simulink model "WindPrototipeN"  (R2019b)
settings: Solver=ode23s  StartTime=0.0  StopTime=Ts  FixedStep=2  RelTol=5
values from neighbouring files (symbols this model uses):
  c1 = 0.51763    [matlab.mat]
  c2 = 116    [matlab.mat]
  c3 = 0.4    [matlab.mat]
  c4 = 5    [matlab.mat]
  c5 = 21    [matlab.mat]
  c6 = 0.006795    [matlab.mat]
  Tp = 2e-05    [matlab.mat]
undefined symbols (not defined in the file or in its folder): Cogent, DiscIntNeverNeededParam, Ion, Kepware, Lithium, localhost, sigbuilder_block
libraries: powerlib x266, powerlib_extras x83, simulink x30, powerlib_meascontrol x13, opclib x11, sldrtlib x8, electricdrivelib x3
(part 1 of 9)
settings Model: SimulationMode=accelerator  NumberOfSteps=100  Creator=cbhende  LastModifiedBy=EK
settings SolverCC: ZeroCrossControl=DisableAll  AutoInsertRateTranBlk=on
settings DataIOCC: LimitDataPoints=on  LoadInitialState=on  SaveFormat=StructureWithTime  SignalLoggingSaveFormat=ModelDataLogs  SaveOutput=off  SignalLogging=off  SaveTime=off  ReturnWorkspaceOutputs=off
settings OptimizationCC: DefaultParameterBehavior=Inlined  ExpressionDepthLimit=2147483647  InitFltsAndDblsToZero=on  EfficientFloat2IntCast=on  LifeSpan=inf
settings DebuggingCC: UnderspecifiedInitializationDetection=Classic  MergeDetectMultiDrivingBlocksExec=none  SolverPrmCheckMsg=warning  MultiTaskRateTransMsg=warning  FcnCallInpInsideContextMsg=warning  StateNameClashWarn=warning  SFUnexpectedBacktrackingDiag=warning  SFNoUnconditionalDefaultTransitionDiag=warning  SFExecutionAtInitializationDiag=none  ArithmeticOperatorsInVariantConditions=warning
settings HardwareCC: ProdBitPerPointer=32  ProdBitPerSizeT=32  ProdBitPerPtrDiffT=32  ProdLargestAtomicFloat=None  ProdIntDivRoundTo=Undefined  ProdEndianess=Unspecified  ProdWordSize=32  ProdHWDeviceType=32-bit Generic
settings ModelReferenceCC: PropagateSignalLabelsOutOfModel=off
settings SFSimCC: SimUseLocalCustomCode=off  CustomCodeUndefinedFunction=UseInterfaceOnly
settings RTWCC: RTWUseLocalCustomCode=off
settings CodeAppCC: StateflowObjectComments=on
settings GRTTargetCC: TargetLangStandard=C89/C90 (ANSI)  GeneratePreprocessorConditionals=Disable all  CombineOutputUpdateFcns=off  GRTInterface=on
settings ConfigComp: CovMetricSettings=dw  CovHtmlReporting=on  CovSaveCumulativeToWorkspaceVar=on  CovSaveSingleToWorkspaceVar=on  CovExternalEMLEnable=off

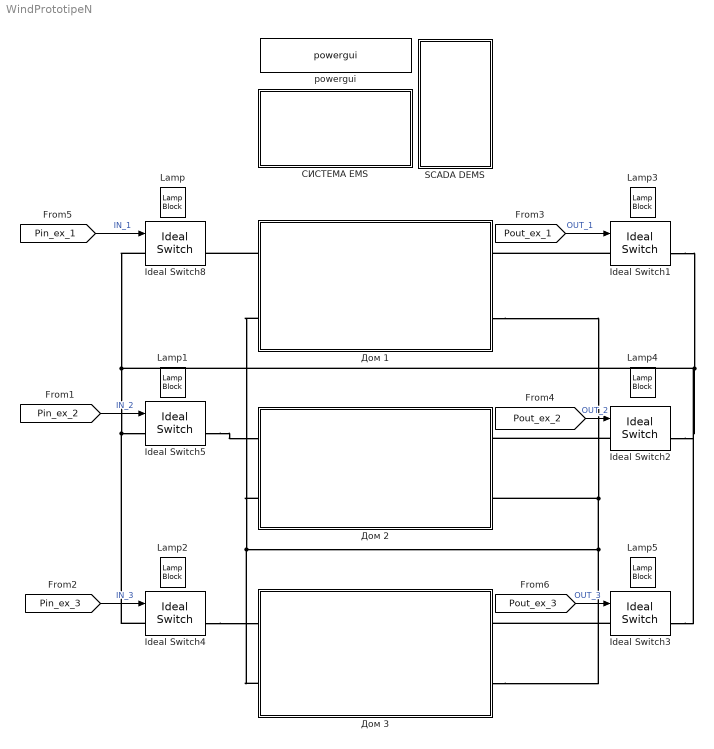
== system WindPrototipeN ==
  Ideal Switch{1..5,8} (6 alike) : powerlib/Power Electronics/Ideal Switch  Ron=0.001  Lon=0  IC=0  Rs=1e5  Cs=inf  Measurements=on
      settings: SourceProductName=Simscape Electrical
  Lamp{,1..5} (6 alike) : LampBlock
  SCADA DEMS : Subsystem
  powergui : powerlib/powergui  Priority=1  SimulationMode=Discrete  SampleTime=Tp  frequency=60  Iterations=50  frequencyindice=0  Pbase=100e6  ErrMax=1e-4  UnitsV=kV  UnitsW=MW  buscounter=0  FunctionMessages=off  echomessages=off  EnableUseOfTLC=off  CurrentSourceSwitches=off  DisableSnubberDevices=off  DisableRonSwitches=off  DisableVfSwitches=off  DisplayEquations=off  AutomaticDiscreteSolvers=off  SolverType=Tustin/Backward Euler (TBE)  Interpol=off  ExternalGateDelay=off  methode=off  Ts=100  x0status=blocks  SPID=off  SwTol=0  HookPort=off  NonlinearTolerance=1e-4  nMaxIteration=100  ContinueOnMaxIteration=off  RestoreLinks=warning  ResistiveCurrentMeasurement=off  Frange=[0:2:500]  Ylog=off  Xlog=on  ShowGrid=off  save=off  variable=ZData  structure=Generator_Terminal  ZoomFFT=off  StartTime=0.0  cycles=1  DisplayStyle=1  fundamental=50  FreqAxis=off  MaxFrequency=4000  frequencyindicesteady=1  RmsSteady=1  display=off
      settings: SourceProductName=Simscape Electrical
  Дом 1 : Subsystem
  Дом 2 : Subsystem
  Дом 3 : Subsystem
  СИСТЕМА EMS : Subsystem
  wires:
  [Pin_ex_1] -> Ideal Switch8/1  "IN_1"
  [Pin_ex_2] -> Ideal Switch5/1  "IN_2"
  [Pin_ex_3] -> Ideal Switch4/1  "IN_3"
  [Pout_ex_1] -> Ideal Switch1/1  "OUT_1"
  [Pout_ex_2] -> Ideal Switch2/1  "OUT_2"
  [Pout_ex_3] -> Ideal Switch3/1  "OUT_3"
  connections:
  Ideal Switch1/LConn1 -- Дом 1/RConn1
  Ideal Switch2/LConn1 -- Дом 2/RConn1
  Ideal Switch5/RConn1 -- Дом 2/LConn1
  Дом 1/LConn1 -- Ideal Switch8/RConn1
  Ideal Switch4/RConn1 -- Дом 3/LConn1
  Ideal Switch1/RConn1 -- Ideal Switch3/RConn1 -- Ideal Switch2/RConn1 -- Ideal Switch4/LConn1 -- Ideal Switch5/LConn1 -- Ideal Switch8/LConn1
  Дом 3/LConn2 -- Дом 3/RConn2 -- Дом 1/RConn2 -- Дом 2/RConn2 -- Дом 1/LConn2 -- Дом 2/LConn2
  Ideal Switch3/LConn1 -- Дом 3/RConn1

== system WindPrototipeN/SCADA DEMS ==
  note: Доступная мощность ВИЭ
      | всех домов (кВт)
  note: Нагрузка
      | PV WP
      | Мощность общая
      | в сети
  note: Потребление всех домов
  note: Нагрузка
      | PV WP
      | Мощность общая
      | в сети
  note: Нагрузка
      | PV WP
      | Мощность общая
      | в сети
  Display{1..14} (14 alike) : DisplayBlock  LabelPosition=Hide  Format=short  Transparency=1
  OPC : Subsystem
  THINGSPEAK : Subsystem
  Мониторинг матлаб : Subsystem

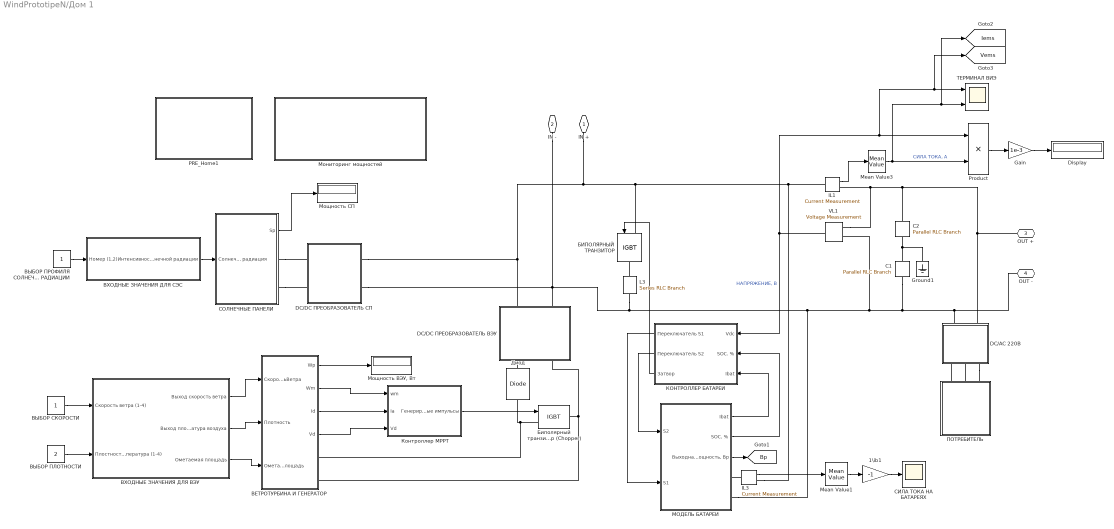
== system WindPrototipeN/Дом 1 ==
  1\ib1 : Gain  Gain=-1  SaturateOnIntegerOverflow=on  OutDataTypeStr=Inherit: Same as input  ParamDataTypeStr=Inherit: Same as input
  C1 : powerlib/Elements/Parallel RLC Branch  LConnTagsString=a  RConnTagsString=__new0  BranchType=C  Resistance=1.0  Inductance=1.0  SetiL0=off  InitialCurrent=0  Capacitance=2200e-06*2  Setx0=off  InitialVoltage=0  Measurements=None
      settings: SourceProductName=Simscape Electrical
  C2 : powerlib/Elements/Parallel RLC Branch  LConnTagsString=a  RConnTagsString=__new0  BranchType=C  Resistance=1.0  Inductance=1.0  SetiL0=off  InitialCurrent=0  Capacitance=2200e-06*2  Setx0=off  InitialVoltage=0  Measurements=None
      settings: SourceProductName=Simscape Electrical
  DC/AC 220В : Subsystem
  DC/DC ПРЕОБРАЗОВАТЕЛЬ ВЭУ : Subsystem
  DC/DC ПРЕОБРАЗОВАТЕЛЬ СП : Subsystem
  Display : Display
  Gain : Gain  Gain=1e-3
  Ground1 : powerlib/Elements/Ground  LConnTagsString=a
      settings: SourceProductName=Simscape Electrical
  IL1 : powerlib/Measurements/Current Measurement  PhasorSimulation=off  OutputType=Complex  PSBequivalent=0
      settings: SourceProductName=Simscape Electrical
  IL3 : powerlib/Measurements/Current Measurement  PhasorSimulation=off  OutputType=Complex  PSBequivalent=0
      settings: SourceProductName=Simscape Electrical
  L3 : powerlib/Elements/Series RLC Branch  LConnTagsString=__new0  RConnTagsString=__new0  BranchType=R  Resistance=19  Inductance=2e-3  SetiL0=off  InitialCurrent=0  Capacitance=1.0  Setx0=off  InitialVoltage=0  Measurements=None
      settings: SourceProductName=Simscape Electrical
  Mean Value1 : powerlib_extras/Measurements/Mean Value  Period=1/110
      settings: SourceProductName=Simscape Electrical  SourceProductBaseCode=PS
  Mean Value3 : powerlib_extras/Measurements/Mean Value  Period=1/110
      settings: SourceProductName=Simscape Electrical  SourceProductBaseCode=PS
  PRE_Home1 : Subsystem
  Product : Product
  VL1 : powerlib/Measurements/Voltage Measurement  Tag=PoWeRsYsTeMmEaSuReMeNt  PhasorSimulation=off  OutputType=Magnitude  PSBequivalent=0
      settings: SourceProductName=Simscape Electrical
  БИПОЛЯРНЫЙ ТРАНЗИТОР : powerlib/Power Electronics/IGBT  Ron=0.001  Lon=0  Vf=1  Tf=1e-6  Tt=2e-6  IC=0  Rs=1e5  Cs=inf  Measurements=off
      settings: SourceProductName=Simscape Electrical
  Биполярный транзистор (Chopper) : powerlib/Power Electronics/IGBT  Ron=0.001  Lon=0  Vf=1  Tf=1e-6  Tt=2e-6  IC=0  Rs=1e5  Cs=inf  Measurements=off
      settings: SourceProductName=Simscape Electrical
  ВЕТРОТУРБИНА И ГЕНЕРАТОР : Subsystem
  ВХОДНЫЕ ЗНАЧЕНИЯ ДЛЯ ВЭУ : Subsystem
  ВХОДНЫЕ ЗНАЧЕНИЯ ДЛЯ СЭС : Subsystem
  ВЫБОР ПЛОТНОСТИ : Constant  Value=2
  ВЫБОР ПРОФИЛЯ СОЛНЕЧНОЙ РАДИАЦИИ : Constant
  ВЫБОР СКОРОСТИ : Constant
  Диод : powerlib/Power Electronics/Diode  Ron=0.01  Lon=0  Vf=0.8  IC=0  UseSnubber=off  Rs=100  Cs=0.1e-6  Measurements=off
      settings: SourceProductName=Simscape Electrical
  КОНТРОЛЛЕР БАТАРЕИ : Subsystem
  Контроллер MPPT : Subsystem
  МОДЕЛЬ БАТАРЕИ : Subsystem
  Мониторинг мощностей : Subsystem
  "Мощность ВЭУ, Вт" : Display
      settings: SampleTime=1e-3
  Мощность СП : Display
      settings: SampleTime=1e-3
  ПОТРЕБИТЕЛЬ : Subsystem
  СИЛА ТОКА НА БАТАРЕЯХ : Scope
  СОЛНЕЧНЫЕ ПАНЕЛИ : Subsystem
  ТЕРМИНАЛ ВИЭ : Scope  NumInputPorts=2
  IN + : PMIOPort  Side=Left
  IN - : PMIOPort  Port=2  Side=Left
  OUT + : PMIOPort  Port=3  Side=Right
  OUT - : PMIOPort  Port=4  Side=Right
  tag scope: Bp=global, Iems=global, Vems=global
  wires:
  1\ib1/1 -> СИЛА ТОКА НА БАТАРЕЯХ/1
  VL1/1 -> КОНТРОЛЛЕР БАТАРЕИ/1(Vdc), [Vems], ТЕРМИНАЛ ВИЭ/1, Product/1  "НАПРЯЖЕНИЕ, В"
  ВЫБОР СКОРОСТИ/1 -> ВХОДНЫЕ ЗНАЧЕНИЯ ДЛЯ ВЭУ/1(Скорость ветра (1-4))
  Mean Value3/1 -> [Iems], ТЕРМИНАЛ ВИЭ/2, Product/2  "СИЛА ТОКА, А"
  МОДЕЛЬ БАТАРЕИ/1(Ibat) -> КОНТРОЛЛЕР БАТАРЕИ/3(Ibat)
  ВХОДНЫЕ ЗНАЧЕНИЯ ДЛЯ ВЭУ/2(Выход плотность и температура воздуха) -> ВЕТРОТУРБИНА И ГЕНЕРАТОР/2(Плотность)
  ВХОДНЫЕ ЗНАЧЕНИЯ ДЛЯ ВЭУ/3(Ометаемая площадь) -> ВЕТРОТУРБИНА И ГЕНЕРАТОР/3(Ометаемая площадь)
  IL1/1 -> Mean Value3/1
  ВЫБОР ПЛОТНОСТИ/1 -> ВХОДНЫЕ ЗНАЧЕНИЯ ДЛЯ ВЭУ/2(Плостность воздуха и температура (1-4))
  IL3/1 -> Mean Value1/1
  Mean Value1/1 -> 1\ib1/1
  ВХОДНЫЕ ЗНАЧЕНИЯ ДЛЯ СЭС/1(Интенсивность солнечной радиации) -> СОЛНЕЧНЫЕ ПАНЕЛИ/1(Солнечная радиация)
  ВХОДНЫЕ ЗНАЧЕНИЯ ДЛЯ ВЭУ/1(Выход скорость ветра) -> ВЕТРОТУРБИНА И ГЕНЕРАТОР/1(СкоростьВетра)
  МОДЕЛЬ БАТАРЕИ/2("SOC, %") -> КОНТРОЛЛЕР БАТАРЕИ/2(SOC. %)
  ВЫБОР ПРОФИЛЯ СОЛНЕЧНОЙ РАДИАЦИИ/1 -> ВХОДНЫЕ ЗНАЧЕНИЯ ДЛЯ СЭС/1(Номер (1,2))
  СОЛНЕЧНЫЕ ПАНЕЛИ/1(Sp) -> Мощность СП/1
  ВЕТРОТУРБИНА И ГЕНЕРАТОР/1(Wp) -> "Мощность ВЭУ, Вт"/1
  Product/1 -> Gain/1
  Gain/1 -> Display/1
  КОНТРОЛЛЕР БАТАРЕИ/2(Переключатель S2) -> МОДЕЛЬ БАТАРЕИ/1(S2)
  КОНТРОЛЛЕР БАТАРЕИ/1(Переключатель S1) -> МОДЕЛЬ БАТАРЕИ/2(S1)
  КОНТРОЛЛЕР БАТАРЕИ/3(Затвор) -> БИПОЛЯРНЫЙ ТРАНЗИТОР/1
  МОДЕЛЬ БАТАРЕИ/3("Выходная мощность, Bp") -> [Bp]
  Контроллер MPPT/1(Генерируемые импульсы) -> Биполярный транзистор (Chopper)/1
  ВЕТРОТУРБИНА И ГЕНЕРАТОР/2(Wm) -> Контроллер MPPT/1(wm)
  ВЕТРОТУРБИНА И ГЕНЕРАТОР/3(Id) -> Контроллер MPPT/2(Ia)
  ВЕТРОТУРБИНА И ГЕНЕРАТОР/4(Vd) -> Контроллер MPPT/3(Vd)
  connections:
  СОЛНЕЧНЫЕ ПАНЕЛИ/RConn2 -- DC/DC ПРЕОБРАЗОВАТЕЛЬ СП/LConn2
  ПОТРЕБИТЕЛЬ/LConn1 -- DC/AC 220В/RConn1
  DC/AC 220В/RConn3 -- ПОТРЕБИТЕЛЬ/LConn3
  Диод/LConn1 -- ВЕТРОТУРБИНА И ГЕНЕРАТОР/RConn1 -- Биполярный транзистор (Chopper)/LConn1
  OUT +/RConn1 -- DC/AC 220В/LConn2 -- C2/LConn1 -- IL1/RConn1 -- VL1/LConn1
  L3/RConn1 -- IN -/RConn1 -- DC/DC ПРЕОБРАЗОВАТЕЛЬ СП/RConn2 -- DC/DC ПРЕОБРАЗОВАТЕЛЬ ВЭУ/RConn2 -- C1/RConn1 -- OUT -/RConn1 -- DC/AC 220В/LConn1 -- VL1/LConn2 -- МОДЕЛЬ БАТАРЕИ/RConn2
  C2/RConn1 -- C1/LConn1 -- Ground1/LConn1
  L3/LConn1 -- БИПОЛЯРНЫЙ ТРАНЗИТОР/RConn1
  ПОТРЕБИТЕЛЬ/LConn2 -- DC/AC 220В/RConn2
  IL3/LConn1 -- МОДЕЛЬ БАТАРЕИ/RConn1
  СОЛНЕЧНЫЕ ПАНЕЛИ/RConn1 -- DC/DC ПРЕОБРАЗОВАТЕЛЬ СП/LConn1
  IL1/LConn1 -- IL3/RConn1 -- DC/DC ПРЕОБРАЗОВАТЕЛЬ ВЭУ/RConn1 -- DC/DC ПРЕОБРАЗОВАТЕЛЬ СП/RConn1 -- IN +/RConn1 -- БИПОЛЯРНЫЙ ТРАНЗИТОР/LConn1
  Биполярный транзистор (Chopper)/RConn1 -- ВЕТРОТУРБИНА И ГЕНЕРАТОР/RConn2 -- DC/DC ПРЕОБРАЗОВАТЕЛЬ ВЭУ/LConn2
  DC/DC ПРЕОБРАЗОВАТЕЛЬ ВЭУ/LConn1 -- Диод/RConn1

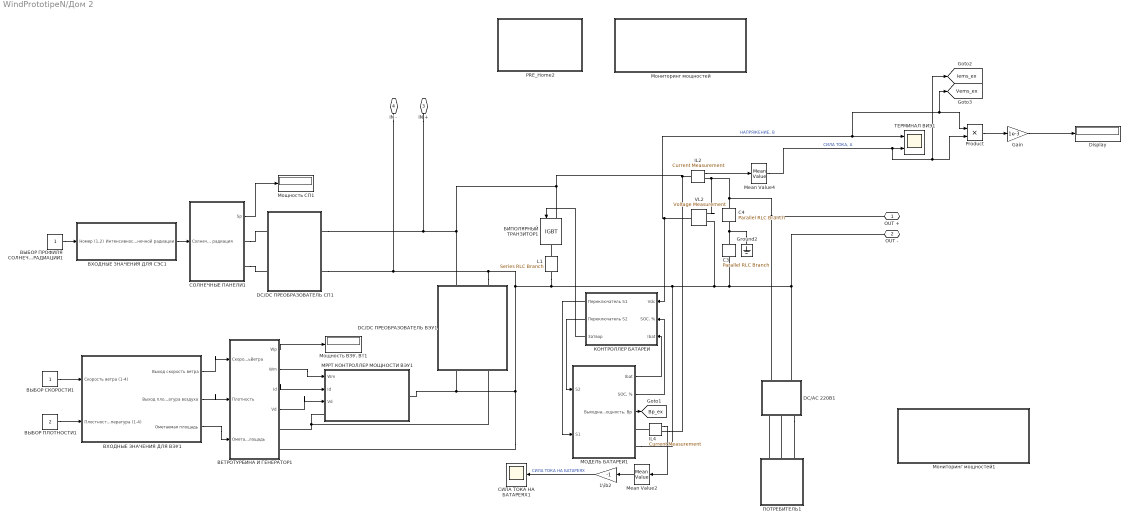
== system WindPrototipeN/Дом 2 ==
  1\ib2 : Gain  Gain=-1  SaturateOnIntegerOverflow=on  OutDataTypeStr=Inherit: Same as input  ParamDataTypeStr=Inherit: Same as input
  C3 : powerlib/Elements/Parallel RLC Branch  LConnTagsString=a  RConnTagsString=__new0  BranchType=C  Resistance=1.0  Inductance=1.0  SetiL0=off  InitialCurrent=0  Capacitance=2200e-06*2  Setx0=off  InitialVoltage=0  Measurements=None
      settings: SourceProductName=Simscape Electrical
  C4 : powerlib/Elements/Parallel RLC Branch  LConnTagsString=a  RConnTagsString=__new0  BranchType=C  Resistance=1.0  Inductance=1.0  SetiL0=off  InitialCurrent=0  Capacitance=2200e-06*2  Setx0=off  InitialVoltage=0  Measurements=None
      settings: SourceProductName=Simscape Electrical
  DC/AC 220В1 : Subsystem
  DC/DC ПРЕОБРАЗОВАТЕЛЬ ВЭУ1 : Subsystem
  DC/DC ПРЕОБРАЗОВАТЕЛЬ СП1 : Subsystem
  Display : Display
  Gain : Gain  Gain=1e-3
  Ground2 : powerlib/Elements/Ground  LConnTagsString=a
      settings: SourceProductName=Simscape Electrical
  IL2 : powerlib/Measurements/Current Measurement  PhasorSimulation=off  OutputType=Complex  PSBequivalent=0
      settings: SourceProductName=Simscape Electrical
  IL4 : powerlib/Measurements/Current Measurement  PhasorSimulation=off  OutputType=Complex  PSBequivalent=0
      settings: SourceProductName=Simscape Electrical
  L1 : powerlib/Elements/Series RLC Branch  LConnTagsString=__new0  RConnTagsString=__new0  BranchType=R  Resistance=19  Inductance=2e-3  SetiL0=off  InitialCurrent=0  Capacitance=1.0  Setx0=off  InitialVoltage=0  Measurements=None
      settings: SourceProductName=Simscape Electrical
  MPPT КОНТРОЛЛЕР МОЩНОСТИ ВЭУ1 : Subsystem
  Mean Value2 : powerlib_extras/Measurements/Mean Value  Period=1/110
      settings: SourceProductName=Simscape Electrical  SourceProductBaseCode=PS
  Mean Value4 : powerlib_extras/Measurements/Mean Value  Period=1/110
      settings: SourceProductName=Simscape Electrical  SourceProductBaseCode=PS
  PRE_Home2 : Subsystem
  Product : Product
  VL2 : powerlib/Measurements/Voltage Measurement  Tag=PoWeRsYsTeMmEaSuReMeNt  PhasorSimulation=off  OutputType=Magnitude  PSBequivalent=0
      settings: SourceProductName=Simscape Electrical
  БИПОЛЯРНЫЙ ТРАНЗИТОР1 : powerlib/Power Electronics/IGBT  Ron=0.001  Lon=0  Vf=1  Tf=1e-6  Tt=2e-6  IC=0  Rs=1e5  Cs=inf  Measurements=off
      settings: SourceProductName=Simscape Electrical
  ВЕТРОТУРБИНА И ГЕНЕРАТОР1 : Subsystem
  ВХОДНЫЕ ЗНАЧЕНИЯ ДЛЯ ВЭУ1 : Subsystem
  ВХОДНЫЕ ЗНАЧЕНИЯ ДЛЯ СЭС1 : Subsystem
  ВЫБОР ПЛОТНОСТИ1 : Constant  Value=2
  ВЫБОР ПРОФИЛЯ СОЛНЕЧНОЙ РАДИАЦИИ1 : Constant
  ВЫБОР СКОРОСТИ1 : Constant
  КОНТРОЛЛЕР БАТАРЕИ : Subsystem
  МОДЕЛЬ БАТАРЕИ1 : Subsystem
  Мониторинг мощностей : Subsystem
  Мониторинг мощностей1 : Subsystem
  "Мощность ВЭУ, Вт1" : Display
      settings: SampleTime=1e-3
  Мощность СП1 : Display
      settings: SampleTime=1e-3
  ПОТРЕБИТЕЛЬ1 : Subsystem
  СИЛА ТОКА НА БАТАРЕЯХ1 : Scope
  СОЛНЕЧНЫЕ ПАНЕЛИ1 : Subsystem
  ТЕРМИНАЛ ВИЭ1 : Scope  NumInputPorts=2
  OUT + : PMIOPort  Side=Right
  OUT - : PMIOPort  Port=2  Side=Right
  IN + : PMIOPort  Port=3  Side=Left
  IN - : PMIOPort  Port=4  Side=Left
  tag scope: Bp_ex=global, Iems_ex=global, Vems_ex=global
  wires:
  1\ib2/1 -> СИЛА ТОКА НА БАТАРЕЯХ1/1  "СИЛА ТОКА НА БАТАРЕЯХ"
  Mean Value2/1 -> 1\ib2/1
  СОЛНЕЧНЫЕ ПАНЕЛИ1/1(Sp) -> Мощность СП1/1
  ВХОДНЫЕ ЗНАЧЕНИЯ ДЛЯ ВЭУ1/2(Выход плотность и температура воздуха) -> ВЕТРОТУРБИНА И ГЕНЕРАТОР1/2(Плотность)
  МОДЕЛЬ БАТАРЕИ1/1(Ibat) -> КОНТРОЛЛЕР БАТАРЕИ/3(Ibat)
  МОДЕЛЬ БАТАРЕИ1/2("SOC, %") -> КОНТРОЛЛЕР БАТАРЕИ/2(SOC. %)
  ВЕТРОТУРБИНА И ГЕНЕРАТОР1/1(Wp) -> "Мощность ВЭУ, Вт1"/1
  ВХОДНЫЕ ЗНАЧЕНИЯ ДЛЯ ВЭУ1/3(Ометаемая площадь) -> ВЕТРОТУРБИНА И ГЕНЕРАТОР1/3(Ометаемая площадь)
  ВЕТРОТУРБИНА И ГЕНЕРАТОР1/3(Id) -> MPPT КОНТРОЛЛЕР МОЩНОСТИ ВЭУ1/2(Id)
  ВХОДНЫЕ ЗНАЧЕНИЯ ДЛЯ СЭС1/1(Интенсивность солнечной радиации) -> СОЛНЕЧНЫЕ ПАНЕЛИ1/1(Солнечная радиация)
  ВЫБОР СКОРОСТИ1/1 -> ВХОДНЫЕ ЗНАЧЕНИЯ ДЛЯ ВЭУ1/1(Скорость ветра (1-4))
  КОНТРОЛЛЕР БАТАРЕИ/1(Переключатель S1) -> МОДЕЛЬ БАТАРЕИ1/2(S1)
  ВЕТРОТУРБИНА И ГЕНЕРАТОР1/2(Wm) -> MPPT КОНТРОЛЛЕР МОЩНОСТИ ВЭУ1/1(Wm)
  ВЫБОР ПРОФИЛЯ СОЛНЕЧНОЙ РАДИАЦИИ1/1 -> ВХОДНЫЕ ЗНАЧЕНИЯ ДЛЯ СЭС1/1(Номер (1,2))
  ВЫБОР ПЛОТНОСТИ1/1 -> ВХОДНЫЕ ЗНАЧЕНИЯ ДЛЯ ВЭУ1/2(Плостность воздуха и температура (1-4))
  ВХОДНЫЕ ЗНАЧЕНИЯ ДЛЯ ВЭУ1/1(Выход скорость ветра) -> ВЕТРОТУРБИНА И ГЕНЕРАТОР1/1(СкоростьВетра)
  КОНТРОЛЛЕР БАТАРЕИ/2(Переключатель S2) -> МОДЕЛЬ БАТАРЕИ1/1(S2)
  IL4/1 -> Mean Value2/1
  IL2/1 -> Mean Value4/1
  КОНТРОЛЛЕР БАТАРЕИ/3(Затвор) -> БИПОЛЯРНЫЙ ТРАНЗИТОР1/1
  ВЕТРОТУРБИНА И ГЕНЕРАТОР1/4(Vd) -> MPPT КОНТРОЛЛЕР МОЩНОСТИ ВЭУ1/3(Vd)
  Product/1 -> Gain/1
  VL2/1 -> [Vems_ex], Product/1, ТЕРМИНАЛ ВИЭ1/1, КОНТРОЛЛЕР БАТАРЕИ/1(Vdc)  "НАПРЯЖЕНИЕ, В"
  Mean Value4/1 -> Product/2, [Iems_ex], ТЕРМИНАЛ ВИЭ1/2  "СИЛА ТОКА, А"
  Gain/1 -> Display/1
  МОДЕЛЬ БАТАРЕИ1/3("Выходная мощность, Bp") -> [Bp_ex]
  connections:
  Ground2/LConn1 -- C4/RConn1 -- C3/LConn1
  VL2/LConn1 -- IL2/RConn1 -- OUT +/RConn1 -- DC/AC 220В1/LConn1 -- C4/LConn1
  DC/DC ПРЕОБРАЗОВАТЕЛЬ ВЭУ1/RConn1 -- DC/DC ПРЕОБРАЗОВАТЕЛЬ СП1/RConn1 -- IN +/RConn1 -- БИПОЛЯРНЫЙ ТРАНЗИТОР1/LConn1 -- IL4/RConn1 -- IL2/LConn1
  IL4/LConn1 -- МОДЕЛЬ БАТАРЕИ1/RConn1
  DC/DC ПРЕОБРАЗОВАТЕЛЬ ВЭУ1/RConn2 -- DC/DC ПРЕОБРАЗОВАТЕЛЬ СП1/RConn2 -- IN -/RConn1 -- МОДЕЛЬ БАТАРЕИ1/RConn2 -- OUT -/RConn1 -- DC/AC 220В1/LConn2 -- C3/RConn1 -- VL2/LConn2 -- L1/RConn1 -- MPPT КОНТРОЛЛЕР МОЩНОСТИ ВЭУ1/RConn1 -- DC/DC ПРЕОБРАЗОВАТЕЛЬ ВЭУ1/LConn1 -- ВЕТРОТУРБИНА И ГЕНЕРАТОР1/RConn2
  DC/DC ПРЕОБРАЗОВАТЕЛЬ ВЭУ1/LConn2 -- MPPT КОНТРОЛЛЕР МОЩНОСТИ ВЭУ1/LConn1 -- ВЕТРОТУРБИНА И ГЕНЕРАТОР1/RConn1
  L1/LConn1 -- БИПОЛЯРНЫЙ ТРАНЗИТОР1/RConn1
  ПОТРЕБИТЕЛЬ1/LConn1 -- DC/AC 220В1/RConn1
  СОЛНЕЧНЫЕ ПАНЕЛИ1/RConn1 -- DC/DC ПРЕОБРАЗОВАТЕЛЬ СП1/LConn1
  ПОТРЕБИТЕЛЬ1/LConn2 -- DC/AC 220В1/RConn2
  DC/AC 220В1/RConn3 -- ПОТРЕБИТЕЛЬ1/LConn3
  СОЛНЕЧНЫЕ ПАНЕЛИ1/RConn2 -- DC/DC ПРЕОБРАЗОВАТЕЛЬ СП1/LConn2

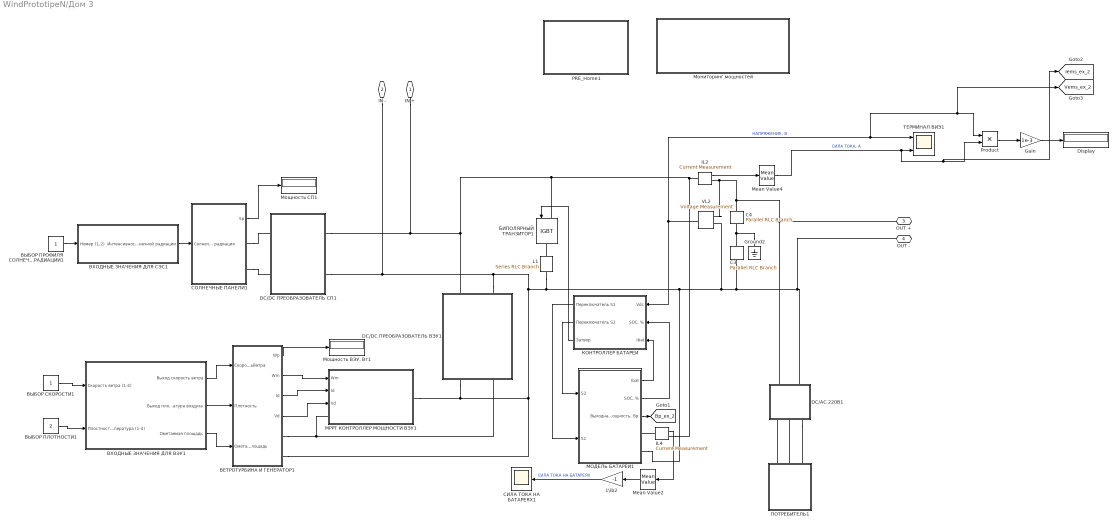
== system WindPrototipeN/Дом 3 ==
  1\ib2 : Gain  Gain=-1  SaturateOnIntegerOverflow=on  OutDataTypeStr=Inherit: Same as input  ParamDataTypeStr=Inherit: Same as input
  C3 : powerlib/Elements/Parallel RLC Branch  LConnTagsString=a  RConnTagsString=__new0  BranchType=C  Resistance=1.0  Inductance=1.0  SetiL0=off  InitialCurrent=0  Capacitance=2200e-06*2  Setx0=off  InitialVoltage=0  Measurements=None
      settings: SourceProductName=Simscape Electrical
  C4 : powerlib/Elements/Parallel RLC Branch  LConnTagsString=a  RConnTagsString=__new0  BranchType=C  Resistance=1.0  Inductance=1.0  SetiL0=off  InitialCurrent=0  Capacitance=2200e-06*2  Setx0=off  InitialVoltage=0  Measurements=None
      settings: SourceProductName=Simscape Electrical
  DC/AC 220В1 : Subsystem
  DC/DC ПРЕОБРАЗОВАТЕЛЬ ВЭУ1 : Subsystem
  DC/DC ПРЕОБРАЗОВАТЕЛЬ СП1 : Subsystem
  Display : Display
  Gain : Gain  Gain=1e-3
  Ground2 : powerlib/Elements/Ground  LConnTagsString=a
      settings: SourceProductName=Simscape Electrical
  IL2 : powerlib/Measurements/Current Measurement  PhasorSimulation=off  OutputType=Complex  PSBequivalent=0
      settings: SourceProductName=Simscape Electrical
  IL4 : powerlib/Measurements/Current Measurement  PhasorSimulation=off  OutputType=Complex  PSBequivalent=0
      settings: SourceProductName=Simscape Electrical
  L1 : powerlib/Elements/Series RLC Branch  LConnTagsString=__new0  RConnTagsString=__new0  BranchType=R  Resistance=19  Inductance=2e-3  SetiL0=off  InitialCurrent=0  Capacitance=1.0  Setx0=off  InitialVoltage=0  Measurements=None
      settings: SourceProductName=Simscape Electrical
  MPPT КОНТРОЛЛЕР МОЩНОСТИ ВЭУ1 : Subsystem
  Mean Value2 : powerlib_extras/Measurements/Mean Value  Period=1/110
      settings: SourceProductName=Simscape Electrical  SourceProductBaseCode=PS
  Mean Value4 : powerlib_extras/Measurements/Mean Value  Period=1/110
      settings: SourceProductName=Simscape Electrical  SourceProductBaseCode=PS
  PRE_Home1 : Subsystem
  Product : Product
  VL2 : powerlib/Measurements/Voltage Measurement  Tag=PoWeRsYsTeMmEaSuReMeNt  PhasorSimulation=off  OutputType=Magnitude  PSBequivalent=0
      settings: SourceProductName=Simscape Electrical
  БИПОЛЯРНЫЙ ТРАНЗИТОР1 : powerlib/Power Electronics/IGBT  Ron=0.001  Lon=0  Vf=1  Tf=1e-6  Tt=2e-6  IC=0  Rs=1e5  Cs=inf  Measurements=off
      settings: SourceProductName=Simscape Electrical
  ВЕТРОТУРБИНА И ГЕНЕРАТОР1 : Subsystem
  ВХОДНЫЕ ЗНАЧЕНИЯ ДЛЯ ВЭУ1 : Subsystem
  ВХОДНЫЕ ЗНАЧЕНИЯ ДЛЯ СЭС1 : Subsystem
  ВЫБОР ПЛОТНОСТИ1 : Constant  Value=2
  ВЫБОР ПРОФИЛЯ СОЛНЕЧНОЙ РАДИАЦИИ1 : Constant
  ВЫБОР СКОРОСТИ1 : Constant
  КОНТРОЛЛЕР БАТАРЕИ : Subsystem
  МОДЕЛЬ БАТАРЕИ1 : Subsystem
  Мониторинг мощностей : Subsystem
  "Мощность ВЭУ, Вт1" : Display
      settings: SampleTime=1e-3
  Мощность СП1 : Display
      settings: SampleTime=1e-3
  ПОТРЕБИТЕЛЬ1 : Subsystem
  СИЛА ТОКА НА БАТАРЕЯХ1 : Scope
  СОЛНЕЧНЫЕ ПАНЕЛИ1 : Subsystem
  ТЕРМИНАЛ ВИЭ1 : Scope  NumInputPorts=2
  IN + : PMIOPort  Side=Left
  IN - : PMIOPort  Port=2  Side=Left
  OUT + : PMIOPort  Port=3  Side=Right
  OUT - : PMIOPort  Port=4  Side=Right
  tag scope: Bp_ex_2=global, Iems_ex_2=global, Vems_ex_2=global
  wires:
  1\ib2/1 -> СИЛА ТОКА НА БАТАРЕЯХ1/1  "СИЛА ТОКА НА БАТАРЕЯХ"
  Mean Value2/1 -> 1\ib2/1
  СОЛНЕЧНЫЕ ПАНЕЛИ1/1(Sp) -> Мощность СП1/1
  ВХОДНЫЕ ЗНАЧЕНИЯ ДЛЯ ВЭУ1/2(Выход плотность и температура воздуха) -> ВЕТРОТУРБИНА И ГЕНЕРАТОР1/2(Плотность)
  МОДЕЛЬ БАТАРЕИ1/1(Ibat) -> КОНТРОЛЛЕР БАТАРЕИ/3(Ibat)
  МОДЕЛЬ БАТАРЕИ1/2("SOC, %") -> КОНТРОЛЛЕР БАТАРЕИ/2(SOC. %)
  ВЕТРОТУРБИНА И ГЕНЕРАТОР1/1(Wp) -> "Мощность ВЭУ, Вт1"/1
  ВХОДНЫЕ ЗНАЧЕНИЯ ДЛЯ ВЭУ1/3(Ометаемая площадь) -> ВЕТРОТУРБИНА И ГЕНЕРАТОР1/3(Ометаемая площадь)
  ВЕТРОТУРБИНА И ГЕНЕРАТОР1/3(Id) -> MPPT КОНТРОЛЛЕР МОЩНОСТИ ВЭУ1/2(Id)
  ВХОДНЫЕ ЗНАЧЕНИЯ ДЛЯ СЭС1/1(Интенсивность солнечной радиации) -> СОЛНЕЧНЫЕ ПАНЕЛИ1/1(Солнечная радиация)
  ВЫБОР СКОРОСТИ1/1 -> ВХОДНЫЕ ЗНАЧЕНИЯ ДЛЯ ВЭУ1/1(Скорость ветра (1-4))
  КОНТРОЛЛЕР БАТАРЕИ/1(Переключатель S1) -> МОДЕЛЬ БАТАРЕИ1/2(S1)
  ВЕТРОТУРБИНА И ГЕНЕРАТОР1/2(Wm) -> MPPT КОНТРОЛЛЕР МОЩНОСТИ ВЭУ1/1(Wm)
  ВЫБОР ПРОФИЛЯ СОЛНЕЧНОЙ РАДИАЦИИ1/1 -> ВХОДНЫЕ ЗНАЧЕНИЯ ДЛЯ СЭС1/1(Номер (1,2))
  ВЫБОР ПЛОТНОСТИ1/1 -> ВХОДНЫЕ ЗНАЧЕНИЯ ДЛЯ ВЭУ1/2(Плостность воздуха и температура (1-4))
  ВХОДНЫЕ ЗНАЧЕНИЯ ДЛЯ ВЭУ1/1(Выход скорость ветра) -> ВЕТРОТУРБИНА И ГЕНЕРАТОР1/1(СкоростьВетра)
  КОНТРОЛЛЕР БАТАРЕИ/2(Переключатель S2) -> МОДЕЛЬ БАТАРЕИ1/1(S2)
  IL4/1 -> Mean Value2/1
  IL2/1 -> Mean Value4/1
  КОНТРОЛЛЕР БАТАРЕИ/3(Затвор) -> БИПОЛЯРНЫЙ ТРАНЗИТОР1/1
  ВЕТРОТУРБИНА И ГЕНЕРАТОР1/4(Vd) -> MPPT КОНТРОЛЛЕР МОЩНОСТИ ВЭУ1/3(Vd)
  Product/1 -> Gain/1
  VL2/1 -> КОНТРОЛЛЕР БАТАРЕИ/1(Vdc), [Vems_ex_2], Product/1, ТЕРМИНАЛ ВИЭ1/1  "НАПРЯЖЕНИЕ, В"
  Mean Value4/1 -> [Iems_ex_2], Product/2, ТЕРМИНАЛ ВИЭ1/2  "СИЛА ТОКА, А"
  Gain/1 -> Display/1
  МОДЕЛЬ БАТАРЕИ1/3("Выходная мощность, Bp") -> [Bp_ex_2]
  connections:
  Ground2/LConn1 -- C4/RConn1 -- C3/LConn1
  VL2/LConn1 -- IL2/RConn1 -- OUT +/RConn1 -- DC/AC 220В1/LConn1 -- C4/LConn1
  IL4/LConn1 -- МОДЕЛЬ БАТАРЕИ1/RConn1
  DC/DC ПРЕОБРАЗОВАТЕЛЬ ВЭУ1/RConn2 -- DC/DC ПРЕОБРАЗОВАТЕЛЬ СП1/RConn2 -- IN -/RConn1 -- ВЕТРОТУРБИНА И ГЕНЕРАТОР1/RConn2 -- DC/DC ПРЕОБРАЗОВАТЕЛЬ ВЭУ1/LConn1 -- MPPT КОНТРОЛЛЕР МОЩНОСТИ ВЭУ1/RConn1 -- МОДЕЛЬ БАТАРЕИ1/RConn2 -- OUT -/RConn1 -- DC/AC 220В1/LConn2 -- C3/RConn1 -- VL2/LConn2 -- L1/RConn1
  L1/LConn1 -- БИПОЛЯРНЫЙ ТРАНЗИТОР1/RConn1
  ПОТРЕБИТЕЛЬ1/LConn1 -- DC/AC 220В1/RConn1
  СОЛНЕЧНЫЕ ПАНЕЛИ1/RConn1 -- DC/DC ПРЕОБРАЗОВАТЕЛЬ СП1/LConn1
  ПОТРЕБИТЕЛЬ1/LConn2 -- DC/AC 220В1/RConn2
  DC/AC 220В1/RConn3 -- ПОТРЕБИТЕЛЬ1/LConn3
  СОЛНЕЧНЫЕ ПАНЕЛИ1/RConn2 -- DC/DC ПРЕОБРАЗОВАТЕЛЬ СП1/LConn2
  ВЕТРОТУРБИНА И ГЕНЕРАТОР1/RConn1 -- MPPT КОНТРОЛЛЕР МОЩНОСТИ ВЭУ1/LConn1 -- DC/DC ПРЕОБРАЗОВАТЕЛЬ ВЭУ1/LConn2
  DC/DC ПРЕОБРАЗОВАТЕЛЬ СП1/RConn1 -- IN +/RConn1 -- DC/DC ПРЕОБРАЗОВАТЕЛЬ ВЭУ1/RConn1 -- IL4/RConn1 -- IL2/LConn1 -- БИПОЛЯРНЫЙ ТРАНЗИТОР1/LConn1

== system WindPrototipeN/СИСТЕМА EMS ==
  Chart3 : Stateflow chart  BlockKeywords=__PRM__SERIALIZED__DATA__:Stateflow Chart,Stateflow Diagram  TreatAsAtomicUnit=on
  Demux : Demux  Outputs=3
  Demux1 : Demux
  Demux2 : Demux
  Demux3 : Demux
  EMS дом 1 : Stateflow chart  BlockKeywords=__PRM__SERIALIZED__DATA__:Stateflow Chart,Stateflow Diagram  TreatAsAtomicUnit=on
  EMS дом 2 : Stateflow chart  BlockKeywords=__PRM__SERIALIZED__DATA__:Stateflow Chart,Stateflow Diagram  TreatAsAtomicUnit=on
  EMS дом 3 : Stateflow chart  BlockKeywords=__PRM__SERIALIZED__DATA__:Stateflow Chart,Stateflow Diagram  TreatAsAtomicUnit=on
  OPC : Subsystem
  Измерение параметров виртуальной станции 1 : Subsystem
  Команды ручного управления дом 1 : opclib/OPC Read  serverHost=localhost  serverID=Kepware.KEPServerEX.V6  itemIDs=Channel1.Device1.Home1.LoadCon, Channel1.Device1.Home1.Pincmd, Channel1.Device1.Home1.Poutcmd, Channel1.Device1.Home1.BatRef  readMode=Asynchronous (device)  dataType=double  updateRate=0.05  showQual=off  showTS=off  tsMode=Seconds since start
      settings: SourceProductName=OPC Toolbox  SourceProductBaseCode=OT
  Команды ручного управления дом 2 : opclib/OPC Read  serverHost=localhost  serverID=Kepware.KEPServerEX.V6  itemIDs=Channel1.Device1.Home2.LoadCon, Channel1.Device1.Home2.Pincmd, Channel1.Device1.Home2.Poutcmd, Channel1.Device1.Home2.BatRef  readMode=Asynchronous (device)  dataType=double  updateRate=0.05  showQual=off  showTS=off  tsMode=Seconds since start
      settings: SourceProductName=OPC Toolbox  SourceProductBaseCode=OT
  Команды ручного управления дом 3 : opclib/OPC Read  serverHost=localhost  serverID=Kepware.KEPServerEX.V6  itemIDs=Channel1.Device1.Home3.LoadCon, Channel1.Device1.Home3.Pincmd, Channel1.Device1.Home3.Poutcmd, Channel1.Device1.Home3.BatRef  readMode=Asynchronous (device)  dataType=double  updateRate=0.05  showQual=off  showTS=off  tsMode=Seconds since start
      settings: SourceProductName=OPC Toolbox  SourceProductBaseCode=OT
  Чтение команд управления : opclib/OPC Read  serverHost=localhost  serverID=Kepware.KEPServerEX.V6  itemIDs=Channel1.Device1.Home1.EMScmd, Channel1.Device1.Home2.EMScmd, Channel1.Device1.Home3.EMScmd  readMode=Asynchronous (device)  dataType=int32  updateRate=0.05  showQual=off  showTS=off  tsMode=Seconds since start
      settings: SourceProductName=OPC Toolbox  SourceProductBaseCode=OT
  станция 2 : Subsystem
  станция 3 : Subsystem
  tag scope: BatCon_ex_1=global, BatCon_ex_2=global, BatCon_ex_3=global, ConLoad_ex_1=global, ConLoad_ex_2=global, ConLoad_ex_3=global, Pin_ex_1=global, Pin_ex_2=global, Pin_ex_3=global, Pout_ex_1=global, Pout_ex_2=global, Pout_ex_3=global
  wires:
  Demux/3 -> EMS дом 3/9(ESS)
  Demux/2 -> EMS дом 2/9(ESS)
  EMS дом 2/4(Ppost) -> OPC/2(In2)
  [HomeC] -> EMS дом 1/8(PpostIN2)
  Измерение параметров виртуальной станции 1/1(<WP>) -> EMS дом 1/1(WP)
  EMS дом 1/2(Pout) -> [Pout_ex_1]
  EMS дом 1/3(Pin) -> [Pin_ex_1]
  Измерение параметров виртуальной станции 1/4(SOC (%)) -> EMS дом 1/4(SOC)
  Измерение параметров виртуальной станции 1/2(<PV>) -> EMS дом 1/2(PV)
  Измерение параметров виртуальной станции 1/5(<Bp>) -> EMS дом 1/5(Bp)
  [HomeB] -> EMS дом 1/7(PpostIN1)
  OPC/1(Out1) -> [HomeA]
  Чтение команд управления/1 -> Demux/1
  EMS дом 3/4(Ppost) -> OPC/3(In3)
  Измерение параметров виртуальной станции 1/3(<Load>) -> EMS дом 1/3(Load)
  EMS дом 1/4(Ppost) -> OPC/1(In1)
  OPC/3(Out3) -> [HomeC]
  EMS дом 1/1(Vbatcmd) -> [BatCon_ex_1]  "Pbatcmd"
  OPC/2(Out2) -> [HomeB]
  Demux/1 -> EMS дом 1/9(ESS)
  EMS дом 1/5(ConnectedLoads) -> [ConLoad_ex_1]
  Команды ручного управления дом 1/1 -> Demux1/1
  Demux1/1 -> EMS дом 1/10(ConnectedLoads_Man)
  Demux1/2 -> EMS дом 1/11(Pin_Man)
  Demux1/3 -> EMS дом 1/12(Pout_Man)
  Demux1/4 -> EMS дом 1/13(Vbatcmd_Man)
  станция 3/1(<WP>) -> EMS дом 3/1(WP)
  станция 3/2(<PV>) -> EMS дом 3/2(PV)
  станция 3/3(<Load>) -> EMS дом 3/3(Load)
  станция 3/4(SOC (%)) -> EMS дом 3/4(SOC)
  станция 3/5(<Bp>) -> EMS дом 3/5(Bp)
  EMS дом 2/5(ConnectedLoads) -> [ConLoad_ex_2]
  EMS дом 2/3(Pin) -> [Pin_ex_2]
  EMS дом 2/2(Pout) -> [Pout_ex_2]
  EMS дом 2/1(Vbatcmd) -> [BatCon_ex_2]  "Pbatcmd"
  EMS дом 3/5(ConnectedLoads) -> [ConLoad_ex_3]
  EMS дом 3/3(Pin) -> [Pin_ex_3]
  EMS дом 3/2(Pout) -> [Pout_ex_3]
  EMS дом 3/1(Vbatcmd) -> [BatCon_ex_3]  "Pbatcmd"
  [HomeA] -> EMS дом 2/7(PpostIN1)
  [HomeC] -> EMS дом 2/8(PpostIN2)
  [HomeB] -> EMS дом 3/7(PpostIN1)
  [HomeA] -> EMS дом 3/8(PpostIN2)
  Demux2/4 -> EMS дом 2/13(Vbatcmd_Man)
  Demux2/2 -> EMS дом 2/11(Pin_Man)
  Demux2/1 -> EMS дом 2/10(ConnectedLoads_Man)
  Demux2/3 -> EMS дом 2/12(Pout_Man)
  Команды ручного управления дом 2/1 -> Demux2/1
  Demux3/4 -> EMS дом 3/13(Vbatcmd_Man)
  Demux3/2 -> EMS дом 3/11(Pin_Man)
  Demux3/1 -> EMS дом 3/10(ConnectedLoads_Man)
  Demux3/3 -> EMS дом 3/12(Pout_Man)
  Команды ручного управления дом 3/1 -> Demux3/1
  Измерение параметров виртуальной станции 1/6(<Bvol>) -> EMS дом 1/6(Bvol)
  станция 2/1(<WP>) -> EMS дом 2/1(WP)
  станция 2/2(<PV>) -> EMS дом 2/2(PV)
  станция 2/3(<Load>) -> EMS дом 2/3(Load)
  станция 2/4(SOC (%)) -> EMS дом 2/4(SOC)
  станция 2/5(<Bp>) -> EMS дом 2/5(Bp)
  станция 2/6(<Bvol>) -> EMS дом 2/6(Bvol)
  станция 3/6(<Bvol>) -> EMS дом 3/6(Bvol)

== system WindPrototipeN/SCADA DEMS/OPC ==
  OPC дом 1 : Subsystem
  OPC дом 2 : Subsystem
  OPC дом 3 : Subsystem
  OPC прочее : Subsystem

== system WindPrototipeN/SCADA DEMS/THINGSPEAK ==
  ThingSpeak Output : sldrtlib/Internet of Things/ThingSpeak Output  DrvAddress=991879  DrvOptions=[1 20 83 48 79 69 86 66 76 71 50 85 52 65 78 51 70 70 97 112 105 46 116 104 105 110 103 115 112 101 97 107 46 99 111 109 0 0 0 0 0 0 0 0 0 0 0 0 0 0 0 0 0 0 0 0 0 0 0 0 0 0 0 0 0 0 0 0 0 0 0 0 0 0 0 0 0 0 0 0 0 0 0 0 0 0 0 0 0 0 0 0 0 0 0 0 0 0 0 0 0 0 0 0 0 0 0 0 0 0 0 0 0 0 0 0 0 0 0 0 0 0 0 0 0 0 0 0 0 0 0 0 0 0 0 0 0 0 0 0 0 0 0 0 0 0 0 0 0 0 0 0 0 0 0 0 0 0 0 0 0 0 0 0 0 0 0 0 0 0 0 0 0 0 0 0 0 0 0 0 0 0 0 0 0 0 0 0 0 0 0 0 0 0 0 0 0 0 0 0 0 0 0 0 0 0 0 0 0 0 0 0 0 0 0 0 0 0 0 0 0 0 0 0 0 0 0 0 0 0 0 0 0 0 0 0 0 0 0 0 0 0 0 0 0 0 0 0 0 0 0 0 0 0 0 0]  SampleTime=0.1  MaxMissedTicks=1000000000000000000000000000000000000000000000000  ShowMissedTicks=off  YieldWhenWaiting=on  ChannelFields=1  OptParam=0  InitialValue=[]  FinalValue=[]
      settings: SourceProductName=Simulink Desktop Real-Time  SourceProductBaseCode=WT
  ThingSpeak Output1 : sldrtlib/Internet of Things/ThingSpeak Output  DrvAddress=991879  DrvOptions=[1 20 83 48 79 69 86 66 76 71 50 85 52 65 78 51 70 70 97 112 105 46 116 104 105 110 103 115 112 101 97 107 46 99 111 109 0 0 0 0 0 0 0 0 0 0 0 0 0 0 0 0 0 0 0 0 0 0 0 0 0 0 0 0 0 0 0 0 0 0 0 0 0 0 0 0 0 0 0 0 0 0 0 0 0 0 0 0 0 0 0 0 0 0 0 0 0 0 0 0 0 0 0 0 0 0 0 0 0 0 0 0 0 0 0 0 0 0 0 0 0 0 0 0 0 0 0 0 0 0 0 0 0 0 0 0 0 0 0 0 0 0 0 0 0 0 0 0 0 0 0 0 0 0 0 0 0 0 0 0 0 0 0 0 0 0 0 0 0 0 0 0 0 0 0 0 0 0 0 0 0 0 0 0 0 0 0 0 0 0 0 0 0 0 0 0 0 0 0 0 0 0 0 0 0 0 0 0 0 0 0 0 0 0 0 0 0 0 0 0 0 0 0 0 0 0 0 0 0 0 0 0 0 0 0 0 0 0 0 0 0 0 0 0 0 0 0 0 0 0 0 0 0 0 0 0]  SampleTime=0.1  MaxMissedTicks=1000000000000000000000000000000000000000000000000  ShowMissedTicks=off  YieldWhenWaiting=on  ChannelFields=2  OptParam=0  InitialValue=[]  FinalValue=[]
      settings: SourceProductName=Simulink Desktop Real-Time  SourceProductBaseCode=WT
  ThingSpeak Output2 : sldrtlib/Internet of Things/ThingSpeak Output  DrvAddress=991879  DrvOptions=[1 20 83 48 79 69 86 66 76 71 50 85 52 65 78 51 70 70 97 112 105 46 116 104 105 110 103 115 112 101 97 107 46 99 111 109 0 0 0 0 0 0 0 0 0 0 0 0 0 0 0 0 0 0 0 0 0 0 0 0 0 0 0 0 0 0 0 0 0 0 0 0 0 0 0 0 0 0 0 0 0 0 0 0 0 0 0 0 0 0 0 0 0 0 0 0 0 0 0 0 0 0 0 0 0 0 0 0 0 0 0 0 0 0 0 0 0 0 0 0 0 0 0 0 0 0 0 0 0 0 0 0 0 0 0 0 0 0 0 0 0 0 0 0 0 0 0 0 0 0 0 0 0 0 0 0 0 0 0 0 0 0 0 0 0 0 0 0 0 0 0 0 0 0 0 0 0 0 0 0 0 0 0 0 0 0 0 0 0 0 0 0 0 0 0 0 0 0 0 0 0 0 0 0 0 0 0 0 0 0 0 0 0 0 0 0 0 0 0 0 0 0 0 0 0 0 0 0 0 0 0 0 0 0 0 0 0 0 0 0 0 0 0 0 0 0 0 0 0 0 0 0 0 0 0 0]  SampleTime=0.1  MaxMissedTicks=1000000000000000000000000000000000000000000000000  ShowMissedTicks=off  YieldWhenWaiting=on  ChannelFields=3  OptParam=0  InitialValue=[]  FinalValue=[]
      settings: SourceProductName=Simulink Desktop Real-Time  SourceProductBaseCode=WT
  ThingSpeak Output3 : sldrtlib/Internet of Things/ThingSpeak Output  DrvAddress=991879  DrvOptions=[1 20 83 48 79 69 86 66 76 71 50 85 52 65 78 51 70 70 97 112 105 46 116 104 105 110 103 115 112 101 97 107 46 99 111 109 0 0 0 0 0 0 0 0 0 0 0 0 0 0 0 0 0 0 0 0 0 0 0 0 0 0 0 0 0 0 0 0 0 0 0 0 0 0 0 0 0 0 0 0 0 0 0 0 0 0 0 0 0 0 0 0 0 0 0 0 0 0 0 0 0 0 0 0 0 0 0 0 0 0 0 0 0 0 0 0 0 0 0 0 0 0 0 0 0 0 0 0 0 0 0 0 0 0 0 0 0 0 0 0 0 0 0 0 0 0 0 0 0 0 0 0 0 0 0 0 0 0 0 0 0 0 0 0 0 0 0 0 0 0 0 0 0 0 0 0 0 0 0 0 0 0 0 0 0 0 0 0 0 0 0 0 0 0 0 0 0 0 0 0 0 0 0 0 0 0 0 0 0 0 0 0 0 0 0 0 0 0 0 0 0 0 0 0 0 0 0 0 0 0 0 0 0 0 0 0 0 0 0 0 0 0 0 0 0 0 0 0 0 0 0 0 0 0 0 0]  SampleTime=0.1  MaxMissedTicks=1000000000000000000000000000000000000000000000000  ShowMissedTicks=off  YieldWhenWaiting=on  ChannelFields=4  OptParam=0  InitialValue=[]  FinalValue=[]
      settings: SourceProductName=Simulink Desktop Real-Time  SourceProductBaseCode=WT
  ThingSpeak Output4 : sldrtlib/Internet of Things/ThingSpeak Output  DrvAddress=991879  DrvOptions=[1 20 83 48 79 69 86 66 76 71 50 85 52 65 78 51 70 70 97 112 105 46 116 104 105 110 103 115 112 101 97 107 46 99 111 109 0 0 0 0 0 0 0 0 0 0 0 0 0 0 0 0 0 0 0 0 0 0 0 0 0 0 0 0 0 0 0 0 0 0 0 0 0 0 0 0 0 0 0 0 0 0 0 0 0 0 0 0 0 0 0 0 0 0 0 0 0 0 0 0 0 0 0 0 0 0 0 0 0 0 0 0 0 0 0 0 0 0 0 0 0 0 0 0 0 0 0 0 0 0 0 0 0 0 0 0 0 0 0 0 0 0 0 0 0 0 0 0 0 0 0 0 0 0 0 0 0 0 0 0 0 0 0 0 0 0 0 0 0 0 0 0 0 0 0 0 0 0 0 0 0 0 0 0 0 0 0 0 0 0 0 0 0 0 0 0 0 0 0 0 0 0 0 0 0 0 0 0 0 0 0 0 0 0 0 0 0 0 0 0 0 0 0 0 0 0 0 0 0 0 0 0 0 0 0 0 0 0 0 0 0 0 0 0 0 0 0 0 0 0 0 0 0 0 0 0]  SampleTime=0.1  MaxMissedTicks=1000000000000000000000000000000000000000000000000  ShowMissedTicks=off  YieldWhenWaiting=on  ChannelFields=5  OptParam=0  InitialValue=[]  FinalValue=[]
      settings: SourceProductName=Simulink Desktop Real-Time  SourceProductBaseCode=WT
  ThingSpeak Output5 : sldrtlib/Internet of Things/ThingSpeak Output  DrvAddress=991879  DrvOptions=[1 20 83 48 79 69 86 66 76 71 50 85 52 65 78 51 70 70 97 112 105 46 116 104 105 110 103 115 112 101 97 107 46 99 111 109 0 0 0 0 0 0 0 0 0 0 0 0 0 0 0 0 0 0 0 0 0 0 0 0 0 0 0 0 0 0 0 0 0 0 0 0 0 0 0 0 0 0 0 0 0 0 0 0 0 0 0 0 0 0 0 0 0 0 0 0 0 0 0 0 0 0 0 0 0 0 0 0 0 0 0 0 0 0 0 0 0 0 0 0 0 0 0 0 0 0 0 0 0 0 0 0 0 0 0 0 0 0 0 0 0 0 0 0 0 0 0 0 0 0 0 0 0 0 0 0 0 0 0 0 0 0 0 0 0 0 0 0 0 0 0 0 0 0 0 0 0 0 0 0 0 0 0 0 0 0 0 0 0 0 0 0 0 0 0 0 0 0 0 0 0 0 0 0 0 0 0 0 0 0 0 0 0 0 0 0 0 0 0 0 0 0 0 0 0 0 0 0 0 0 0 0 0 0 0 0 0 0 0 0 0 0 0 0 0 0 0 0 0 0 0 0 0 0 0 0]  SampleTime=0.1  MaxMissedTicks=1000000000000000000000000000000000000000000000000  ShowMissedTicks=off  YieldWhenWaiting=on  ChannelFields=6  OptParam=0  InitialValue=[]  FinalValue=[]
      settings: SourceProductName=Simulink Desktop Real-Time  SourceProductBaseCode=WT
  ThingSpeak Output6 : sldrtlib/Internet of Things/ThingSpeak Output  DrvAddress=991879  DrvOptions=[1 20 83 48 79 69 86 66 76 71 50 85 52 65 78 51 70 70 97 112 105 46 116 104 105 110 103 115 112 101 97 107 46 99 111 109 0 0 0 0 0 0 0 0 0 0 0 0 0 0 0 0 0 0 0 0 0 0 0 0 0 0 0 0 0 0 0 0 0 0 0 0 0 0 0 0 0 0 0 0 0 0 0 0 0 0 0 0 0 0 0 0 0 0 0 0 0 0 0 0 0 0 0 0 0 0 0 0 0 0 0 0 0 0 0 0 0 0 0 0 0 0 0 0 0 0 0 0 0 0 0 0 0 0 0 0 0 0 0 0 0 0 0 0 0 0 0 0 0 0 0 0 0 0 0 0 0 0 0 0 0 0 0 0 0 0 0 0 0 0 0 0 0 0 0 0 0 0 0 0 0 0 0 0 0 0 0 0 0 0 0 0 0 0 0 0 0 0 0 0 0 0 0 0 0 0 0 0 0 0 0 0 0 0 0 0 0 0 0 0 0 0 0 0 0 0 0 0 0 0 0 0 0 0 0 0 0 0 0 0 0 0 0 0 0 0 0 0 0 0 0 0 0 0 0 0]  SampleTime=0.1  MaxMissedTicks=1000000000000000000000000000000000000000000000000  ShowMissedTicks=off  YieldWhenWaiting=on  ChannelFields=8  OptParam=0  InitialValue=[]  FinalValue=[]
      settings: SourceProductName=Simulink Desktop Real-Time  SourceProductBaseCode=WT
  ThingSpeak Output7 : sldrtlib/Internet of Things/ThingSpeak Output  DrvAddress=991879  DrvOptions=[1 20 83 48 79 69 86 66 76 71 50 85 52 65 78 51 70 70 97 112 105 46 116 104 105 110 103 115 112 101 97 107 46 99 111 109 0 0 0 0 0 0 0 0 0 0 0 0 0 0 0 0 0 0 0 0 0 0 0 0 0 0 0 0 0 0 0 0 0 0 0 0 0 0 0 0 0 0 0 0 0 0 0 0 0 0 0 0 0 0 0 0 0 0 0 0 0 0 0 0 0 0 0 0 0 0 0 0 0 0 0 0 0 0 0 0 0 0 0 0 0 0 0 0 0 0 0 0 0 0 0 0 0 0 0 0 0 0 0 0 0 0 0 0 0 0 0 0 0 0 0 0 0 0 0 0 0 0 0 0 0 0 0 0 0 0 0 0 0 0 0 0 0 0 0 0 0 0 0 0 0 0 0 0 0 0 0 0 0 0 0 0 0 0 0 0 0 0 0 0 0 0 0 0 0 0 0 0 0 0 0 0 0 0 0 0 0 0 0 0 0 0 0 0 0 0 0 0 0 0 0 0 0 0 0 0 0 0 0 0 0 0 0 0 0 0 0 0 0 0 0 0 0 0 0 0]  SampleTime=0.1  MaxMissedTicks=1000000000000000000000000000000000000000000000000  ShowMissedTicks=off  YieldWhenWaiting=on  ChannelFields=7  OptParam=0  InitialValue=[]  FinalValue=[]
      settings: SourceProductName=Simulink Desktop Real-Time  SourceProductBaseCode=WT
  wires:
  [LoadHome1] -> ThingSpeak Output4/1
  [SolarPower] -> ThingSpeak Output3/1
  [SolarRad] -> ThingSpeak Output2/1
  [WindPower] -> ThingSpeak Output1/1
  [WindSpeed] -> ThingSpeak Output/1
  [Bsoc] -> ThingSpeak Output5/1
  [Iems] -> ThingSpeak Output6/1
  [Vems] -> ThingSpeak Output7/1

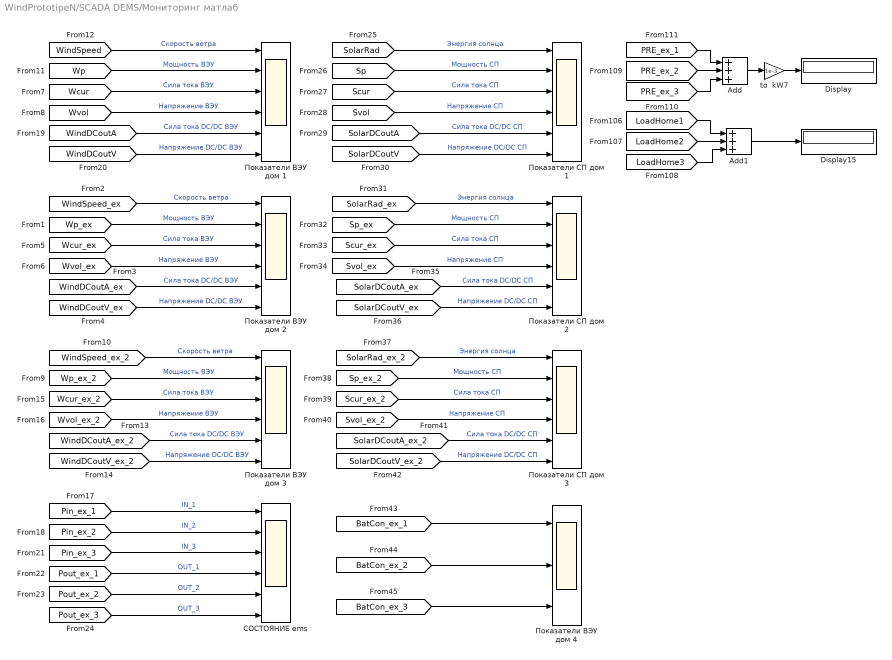
== system WindPrototipeN/SCADA DEMS/Мониторинг матлаб ==
  Add : Sum  Inputs=+++
  Add1 : Sum  Inputs=+++
  Display : Display
  Display15 : Display
  to  kW7 : Gain  Gain=1e-3
  Показатели ВЭУ дом 1 : Scope  NumInputPorts=6
  Показатели ВЭУ дом 2 : Scope  NumInputPorts=6
  Показатели ВЭУ дом 3 : Scope  NumInputPorts=6
  Показатели ВЭУ дом 4 : Scope  NumInputPorts=3
  Показатели СП дом 1 : Scope  NumInputPorts=6
  Показатели СП дом 2 : Scope  NumInputPorts=6
  Показатели СП дом 3 : Scope  NumInputPorts=6
  СОСТОЯНИЕ ems : Scope  NumInputPorts=6
  wires:
  [BatCon_ex_3] -> Показатели ВЭУ дом 4/3
  [WindDCoutA_ex_2] -> Показатели ВЭУ дом 3/5  "Сила тока DC/DC ВЭУ"
  [SolarDCoutV] -> Показатели СП дом 1/6  "Напряжение DC/DC СП"
  [WindDCoutA_ex] -> Показатели ВЭУ дом 2/5  "Сила тока DC/DC ВЭУ"
  [Wp] -> Показатели ВЭУ дом 1/2  "Мощность ВЭУ"
  [SolarDCoutV_ex] -> Показатели СП дом 2/6  "Напряжение DC/DC СП"
  [WindSpeed_ex] -> Показатели ВЭУ дом 2/1  "Скорость ветра"
  [Wcur_ex] -> Показатели ВЭУ дом 2/3  "Сила тока ВЭУ"
  [WindDCoutV_ex] -> Показатели ВЭУ дом 2/6  "Напряжение DC/DC ВЭУ"
  [Wp_ex_2] -> Показатели ВЭУ дом 3/2  "Мощность ВЭУ"
  [WindDCoutV] -> Показатели ВЭУ дом 1/6  "Напряжение DC/DC ВЭУ"
  [BatCon_ex_1] -> Показатели ВЭУ дом 4/1
  [SolarDCoutV_ex_2] -> Показатели СП дом 3/6  "Напряжение DC/DC СП"
  [SolarRad_ex] -> Показатели СП дом 2/1  "Энергия солнца"
  [Wvol_ex] -> Показатели ВЭУ дом 2/4  "Напряжение ВЭУ"
  [Wvol_ex_2] -> Показатели ВЭУ дом 3/4  "Напряжение ВЭУ"
  [WindSpeed] -> Показатели ВЭУ дом 1/1  "Скорость ветра"
  [Wcur_ex_2] -> Показатели ВЭУ дом 3/3  "Сила тока ВЭУ"
  [WindSpeed_ex_2] -> Показатели ВЭУ дом 3/1  "Скорость ветра"
  [SolarDCoutA_ex_2] -> Показатели СП дом 3/5  "Сила тока DC/DC СП"
  [SolarRad] -> Показатели СП дом 1/1  "Энергия солнца"
  [Wp_ex] -> Показатели ВЭУ дом 2/2  "Мощность ВЭУ"
  [Sp_ex_2] -> Показатели СП дом 3/2  "Мощность СП"
  [Pout_ex_2] -> СОСТОЯНИЕ ems/5  "OUT_2"
  [WindDCoutV_ex_2] -> Показатели ВЭУ дом 3/6  "Напряжение DC/DC ВЭУ"
  [Sp] -> Показатели СП дом 1/2  "Мощность СП"
  [Pin_ex_3] -> СОСТОЯНИЕ ems/3  "IN_3"
  [BatCon_ex_2] -> Показатели ВЭУ дом 4/2
  [Pin_ex_2] -> СОСТОЯНИЕ ems/2  "IN_2"
  [Svol] -> Показатели СП дом 1/4  "Напряжение СП"
  [Scur] -> Показатели СП дом 1/3  "Сила тока СП"
  [Pout_ex_3] -> СОСТОЯНИЕ ems/6  "OUT_3"
  [Wvol] -> Показатели ВЭУ дом 1/4  "Напряжение ВЭУ"
  [Wcur] -> Показатели ВЭУ дом 1/3  "Сила тока ВЭУ"
  [Sp_ex] -> Показатели СП дом 2/2  "Мощность СП"
  [WindDCoutA] -> Показатели ВЭУ дом 1/5  "Сила тока DC/DC ВЭУ"
  [Svol_ex] -> Показатели СП дом 2/4  "Напряжение СП"
  [Pin_ex_1] -> СОСТОЯНИЕ ems/1  "IN_1"
  [Pout_ex_1] -> СОСТОЯНИЕ ems/4  "OUT_1"
  [SolarDCoutA] -> Показатели СП дом 1/5  "Сила тока DC/DC СП"
  [SolarDCoutA_ex] -> Показатели СП дом 2/5  "Сила тока DC/DC СП"
  [Svol_ex_2] -> Показатели СП дом 3/4  "Напряжение СП"
  [Scur_ex_2] -> Показатели СП дом 3/3  "Сила тока СП"
  [Scur_ex] -> Показатели СП дом 2/3  "Сила тока СП"
  [SolarRad_ex_2] -> Показатели СП дом 3/1  "Энергия солнца"
  [PRE_ex_2] -> Add/2
  to  kW7/1 -> Display/1
  [PRE_ex_3] -> Add/3
  Add/1 -> to  kW7/1
  [LoadHome3] -> Add1/3
  Add1/1 -> Display15/1
  [LoadHome1] -> Add1/1
  [PRE_ex_1] -> Add/1
  [LoadHome2] -> Add1/2

== system WindPrototipeN/Дом 1/DC//AC 220В ==
  LC Фильтр : Subsystem
  PWM IGBT Inverter1 : powerlib/Power Electronics/Universal Bridge  Arms=3  SnubberResistance=5000  SnubberCapacitance=inf  Device=IGBT / Diodes  Ron=1e-3  Lon=0  ForwardVoltages="[  0.0  0.0  ]"  ForwardVoltage=.8  GTOparameters=[ 1e-6 ,1e-6 ]  IGBTparameters=[ 1e-6 , 2e-6 ]  Measurements=Device currents  Measurements_2=None  converterType=Rectifier
      settings: SourceProductName=Simscape Electrical
  Инвертор DC/AC : Subsystem
  Терминал инвертора : Scope  NumInputPorts=2
  A : PMIOPort  Side=Right
  B : PMIOPort  Port=2  Side=Right
  C : PMIOPort  Port=3  Side=Right
  - IGBT1 : PMIOPort  Port=4  Side=Left
  + IGBT1 : PMIOPort  Port=5  Side=Left
  tag scope: Vgrid=global
  wires:
  Инвертор DC/AC/3(Pulses) -> PWM IGBT Inverter1/1
  Инвертор DC/AC/1(VL) -> Терминал инвертора/1  "Напряжение на входе, В"
  Инвертор DC/AC/2(Vp) -> [Vgrid], Терминал инвертора/2  "Напряжение от преобразователя, В"
  connections:
  LC Фильтр/LConn1 -- PWM IGBT Inverter1/LConn1
  LC Фильтр/RConn3 -- C/RConn1 -- Инвертор DC/AC/LConn1
  Инвертор DC/AC/LConn2 -- B/RConn1 -- LC Фильтр/RConn2
  LC Фильтр/RConn1 -- A/RConn1 -- Инвертор DC/AC/LConn3
  LC Фильтр/LConn3 -- PWM IGBT Inverter1/LConn3
  LC Фильтр/LConn2 -- PWM IGBT Inverter1/LConn2
  + IGBT1/RConn1 -- PWM IGBT Inverter1/RConn1
  - IGBT1/RConn1 -- PWM IGBT Inverter1/RConn2

== system WindPrototipeN/Дом 1/DC//DC ПРЕОБРАЗОВАТЕЛЬ ВЭУ ==
  Add : Sum
  CBus : powerlib/Elements/Series RLC Branch  LConnTagsString=__new0  RConnTagsString=__new0  BranchType=RC  Resistance=0.2  Inductance=1e-3  SetiL0=off  InitialCurrent=0  Capacitance=7500e-6  Setx0=on  InitialVoltage=100  Measurements=None
      settings: SourceProductName=Simscape Electrical
  Chopper : Subsystem  mask(SPSdrives Converter){SnubberResistance=10e3, SnubberCapacitance=inf, Ron=1e-3, ForwardVoltages=[1.3,1.3], IGBTParameters=[0,0], converterType=Inverter}
      mask prompts: SnubberResistance "Snubber resistance Rs (Ohms):"; SnubberCapacitance "Snubber capacitance Cs (F):"; Ron "Ron (Ohms):"; ForwardVoltages "Forward voltages [Device Vf(V), Diode Vd (V)]"; IGBTParameters "[Tf(s), Tt(s)]:"; converterType "Converter type:"
      mask help: This model implements an average-value buck converter."Duty Cycle" contains the duty cycle of the internal IGBT device.
      mask TypeOptions converterType: Rectifier | Inverter
      mask Display: plot(0,0,100,100,[39 39 23.8],[71 28 28],[44 56 49.6 56 52.8 56 61 61],[39.2 33.6 32.8 33.6 40.8 33.6 30 12.4],[44 44 44 61 61],[28 71 60 66.4 90],[75 67 83 75 67 83 75 75],[54 42 42 54 54 54 54 66],[61 75 75],[24 24 42],[75 75 61],[66,76,76])
  Constant : Constant  Value=100
  Current controller DISCRETE1 : Subsystem  mask(PI controller){Kp=0.0005, Ki=0.15, Ts=20e-6}
      mask prompts: Kp "Proportional gain (Kp)"; Ki "Integral gain (Ki)"; Ts "Sample time (s) :"
      mask help: Proportional-Integral Speed Controller
      mask Display: plot(0,0,100,100,[35,35,65],[70,30,30],[35,65],[45,60])
  Current controller DISCRETE2 : Subsystem  mask(PI controller){Kp=0.0005, Ki=0.15, Ts=20e-6}
      mask prompts: Kp "Proportional gain (Kp)"; Ki "Integral gain (Ki)"; Ts "Sample time (s) :"
      mask help: Proportional-Integral Speed Controller
      mask Display: plot(0,0,100,100,[35,35,65],[70,30,30],[35,65],[45,60])
  Duty Cycles : Subsystem
  IL2 : powerlib/Measurements/Current Measurement  PhasorSimulation=off  OutputType=Complex  PSBequivalent=0
      settings: SourceProductName=Simscape Electrical
  IL4 : powerlib/Measurements/Current Measurement  PhasorSimulation=off  OutputType=Complex  PSBequivalent=0
      settings: SourceProductName=Simscape Electrical
  L : powerlib/Elements/Series RLC Branch  LConnTagsString=__new0  RConnTagsString=__new0  BranchType=L  Resistance=0.3  Inductance=500e-6  SetiL0=off  InitialCurrent=0  Capacitance=100e-6  Setx0=off  InitialVoltage=0  Measurements=None
      settings: SourceProductName=Simscape Electrical
  Timer : Subsystem  DialogController=POWERSYS.PowerSysDialog  mask(Timer){t=[ 0  1], e=[1 1 ]}
      mask prompts: t "Time (s):"; e "Amplitude:"
      mask help:
      | Generates a signal changing at specified times.
      |
      | If a signal value is not specified at time zero, the output is kept at 0 until the first specified transition time.
      mask init:
      | tt=t;
      | sv=e;
      | if isempty(tt) | isempty(sv)
      | 	% probably during the load process when under a masked block.
      | 	tt=0;
      | 	sv=1;
      | end
      | %
      | if length(sv) ~= length(tt),
      |    Erreur.message = 'The vectors specifying the time and amplitude pairs must have the same length.';
      |    Erreur.identifier = 'SimPowerSystems:TimerBlock:ParameterError';
      |    powericon('psberror',Erreur.message,Erreur.identifier,'NoUiwait');
      | end
      | if tt(1)~=0,
      |    tt=[0 tt];
      |    sv=[~sv(1) sv];
      | end
      | n=length(tt);
      | vec_dt=[tt,0]-[0,tt] ;
      | vec_dt=vec_dt(2:n);
      | if any(vec_dt<=0)
      |    Erreur.message = 'All transition times must be in increasing order.';
      |    Erreur.identifier = 'SimPowerSystems:TimerBlock:ParameterError';
      |    powericon('psberror',Erreur.message,Erreur.identifier,'NoUiwait');
      | end
      | tv=[-1,tt(1),reshape(repmat(reshape(tt(2:end),1,length(tt)-1),2,1),1,2*length(tt)-2),tt(end)+1];
      | %sv=(sv(:)'~=0);
      | opv=[sv(1),reshape(repmat(sv(1:end-1),2,1),1,2*length(sv)-2),sv(end),sv(end)];
      | 
      | power_initmask();
      mask Help: web(psbhelp)
      mask Display: plot( tv(2:end-1), opv(2:end-1) )
  Voltage Measurement : powerlib/Measurements/Voltage Measurement  PhasorSimulation=off  OutputType=Complex  PSBequivalent=0
      settings: SourceProductName=Simscape Electrical
  Voltage Measurement1 : powerlib/Measurements/Voltage Measurement  PhasorSimulation=off  OutputType=Complex  PSBequivalent=0
      settings: SourceProductName=Simscape Electrical
  Диод : powerlib/Power Electronics/Diode  Ron=0.01  Lon=0  Vf=0.8  IC=0  UseSnubber=off  Rs=100  Cs=0.1e-6  Measurements=off
      settings: SourceProductName=Simscape Electrical
  Терминал вход : Scope  NumInputPorts=2
  Терминал выход boost DC/DC : Scope  NumInputPorts=2
  Фильтр : TransferFcn  Denominator=[0.001 1]
  Выход + : PMIOPort  Side=Right
  Вход - : PMIOPort  Port=2  Side=Left
  Выход - : PMIOPort  Port=3  Side=Right
  Вход + : PMIOPort  Port=4  Side=Left
  tag scope: WindDCoutA=global, WindDCoutV=global
  wires:
  Duty Cycles/1(dc) -> Chopper/1(Duty Cycle)
  Current controller DISCRETE2/1(Delta Ec) -> Add/2
  Current controller DISCRETE1/1(Ec) -> Add/1
  Voltage Measurement1/1 -> Терминал вход/1
  [Wp] -> Current controller DISCRETE2/2(Ppv)
  IL4/1 -> [WindDCoutA], Терминал выход boost DC/DC/2  "Сила тока, А"
  IL2/1 -> Терминал вход/2  "Сила тока, А"
  Add/1 -> Duty Cycles/1(Ec)
  Timer/1(Out) -> Current controller DISCRETE2/1(Pref)
  Voltage Measurement/1 -> [WindDCoutV], Терминал выход boost DC/DC/1, Фильтр/1
  Constant/1 -> Current controller DISCRETE1/2(Uref)
  Фильтр/1 -> Current controller DISCRETE1/1(UBus)
  connections:
  Voltage Measurement1/LConn1 -- L/RConn1 -- IL2/RConn1
  Chopper/LConn2 -- Вход -/RConn1 -- Voltage Measurement1/LConn2 -- Voltage Measurement/LConn2 -- Выход -/RConn1 -- CBus/RConn1
  IL4/RConn1 -- Выход +/RConn1
  CBus/LConn1 -- IL4/LConn1 -- Voltage Measurement/LConn1 -- Chopper/LConn1
  Вход +/RConn1 -- Диод/LConn1
  Chopper/RConn1 -- L/LConn1
  Диод/RConn1 -- IL2/LConn1
